simulink model "Flat_Robot"  (R2020a)
settings: Solver=VariableStepAuto  StartTime=0.0  StopTime=20  RelTol=1e-3
PostLoadFcn:
  | m=2.5;
  | k_drag=30;
  | r=0.15;
settings Model: Creator=NIKITA  LastModifiedBy=NIKITA

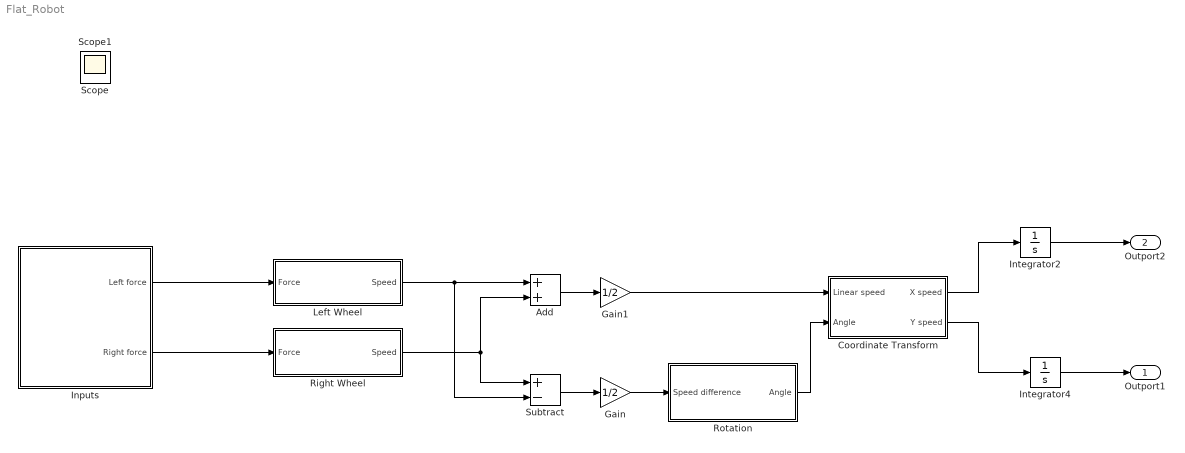
== system Flat_Robot ==
  Add : Sum
  Coordinate Transform : Subsystem
  Gain : Gain  Gain=1/2
  Gain1 : Gain  Gain=1/2
  Inputs : Subsystem
  Integrator2 : Integrator
  Integrator4 : Integrator
  Left Wheel : Subsystem
  Right Wheel : Subsystem
  Rotation : Subsystem
  Subtract : Sum  Inputs=+-
  "Outport1 " : Outport
  "Outport2 " : Outport  Port=2
  Scope : Scope
  Scope1 : Scope
  wires:
  Inputs/2(Right force) -> Right Wheel/1(Force)
  Inputs/1(Left force) -> Left Wheel/1(Force)
  Add/1 -> Gain1/1
  Right Wheel/1(Speed) -> Subtract/1, Add/2
  Left Wheel/1(Speed) -> Subtract/2, Add/1
  Subtract/1 -> Gain/1
  Gain/1 -> Rotation/1(Speed difference)
  Integrator4/1 -> "Outport1 "/1
  Integrator2/1 -> "Outport2 "/1
  Coordinate Transform/1(X speed) -> Integrator2/1
  Coordinate Transform/2(Y speed) -> Integrator4/1
  Rotation/1(Angle) -> Coordinate Transform/2(Angle)
  Gain1/1 -> Coordinate Transform/1(Linear speed)

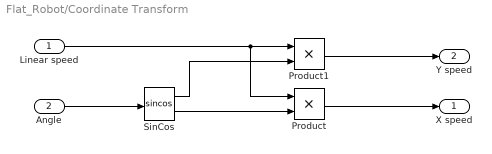
== system Flat_Robot/Coordinate Transform ==
  Linear speed : Inport
  Angle : Inport  Port=2
  Product : Product
  Product1 : Product
  SinCos : Trigonometry  Operator=sincos
  X speed : Outport  VectorParamsAs1DForOutWhenUnconnected=off
  Y speed : Outport  Port=2  VectorParamsAs1DForOutWhenUnconnected=off
  wires:
  Product/1 -> X speed/1
  Product1/1 -> Y speed/1
  Angle/1 -> SinCos/1
  SinCos/1 -> Product1/2
  Linear speed/1 -> Product1/1, Product/1
  SinCos/2 -> Product/2

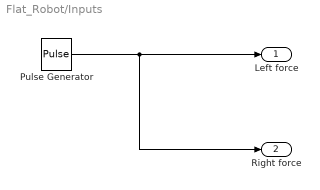
== system Flat_Robot/Inputs ==
  Pulse Generator : DiscretePulseGenerator  PulseType=Time based  Period=20  PulseWidth=15
  Left force : Outport  VectorParamsAs1DForOutWhenUnconnected=off
  Right force : Outport  Port=2  VectorParamsAs1DForOutWhenUnconnected=off
  wires:
  Pulse Generator/1 -> Right force/1, Left force/1

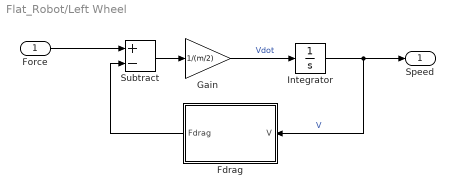
== system Flat_Robot/Left Wheel ==
  Force : Inport
  Fdrag : MATLAB Function  TreatAsAtomicUnit=on
  Gain : Gain  Gain=1/(m/2)
  Integrator : Integrator
  Subtract : Sum  Inputs=+-
  Speed : Outport  VectorParamsAs1DForOutWhenUnconnected=off
  wires:
  Force/1 -> Subtract/1
  Subtract/1 -> Gain/1
  Gain/1 -> Integrator/1  "Vdot"
  Integrator/1 -> Speed/1, Fdrag/1(V)  "V"
  Fdrag/1(Fdrag) -> Subtract/2

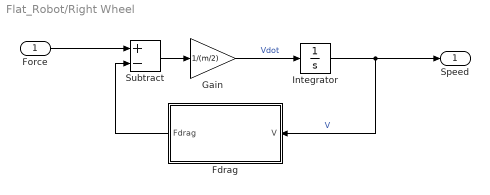
== system Flat_Robot/Right Wheel ==
  Force : Inport
  Fdrag : MATLAB Function  TreatAsAtomicUnit=on
  Gain : Gain  Gain=1/(m/2)
  Integrator : Integrator
  Subtract : Sum  Inputs=+-
  Speed : Outport  VectorParamsAs1DForOutWhenUnconnected=off
  wires:
  Fdrag/1(Fdrag) -> Subtract/2
  Integrator/1 -> Speed/1, Fdrag/1(V)  "V"
  Gain/1 -> Integrator/1  "Vdot"
  Subtract/1 -> Gain/1
  Force/1 -> Subtract/1

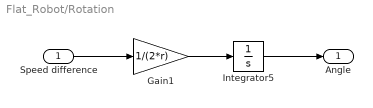
== system Flat_Robot/Rotation ==
  Speed difference : Inport
  Gain1 : Gain  Gain=1/(2*r)
  Integrator5 : Integrator
  Angle : Outport  VectorParamsAs1DForOutWhenUnconnected=off
  wires:
  Speed difference/1 -> Gain1/1
  Gain1/1 -> Integrator5/1
  Integrator5/1 -> Angle/1

== matlab function Flat_Robot/Right Wheel/Fdrag ==
  data: V input; Fdrag output; k_drag parameter
function Fdrag = get_fdrag(V,k_drag)

Fdrag = k_drag*V*abs(V);

== matlab function Flat_Robot/Left Wheel/Fdrag ==
  data: V input; Fdrag output; k_drag parameter
function Fdrag = get_fdrag(V,k_drag)

Fdrag = k_drag*V*abs(V);
